simulink model "Control2_exec_time_sampling_time"  (R2023b)
settings: Solver=ode45  StartTime=0.0  StopTime=inf  RelTol=1e-3  EnableMultiTasking=on
libraries: instrumentseriallib x3
settings Model: Creator=fvg  LastModifiedBy=Usuario
settings SolverCC: AlgebraicLoopSolver=TrustRegion
settings DataIOCC: LimitDataPoints=on  SaveFormat=Array  SignalLoggingSaveFormat=ModelDataLogs  SaveTime=off  ReturnWorkspaceOutputs=off
settings OptimizationCC: ExpressionDepthLimit=2147483647  LifeSpan=inf
settings DebuggingCC: UnderspecifiedInitializationDetection=Classic  MergeDetectMultiDrivingBlocksExec=none  SolverPrmCheckMsg=warning  FcnCallInpInsideContextMsg=warning  UnconnectedInputMsg=warning  UnconnectedOutputMsg=warning  UnconnectedLineMsg=warning  StateNameClashWarn=warning  SFUnexpectedBacktrackingDiag=warning  SFNoUnconditionalDefaultTransitionDiag=warning  SFExecutionAtInitializationDiag=none  ArithmeticOperatorsInVariantConditions=warning
settings HardwareCC: ProdBitPerPointer=32  ProdBitPerSizeT=32  ProdBitPerPtrDiffT=32  ProdLargestAtomicFloat=None  ProdIntDivRoundTo=Undefined  ProdEndianess=Unspecified  ProdWordSize=32  ProdHWDeviceType=32-bit Generic
settings ModelReferenceCC: EnableRefExpFcnMdlSchedulingChecks=on  PropagateSignalLabelsOutOfModel=off
settings SFSimCC: SimUseLocalCustomCode=off  CustomCodeUndefinedFunction=UseInterfaceOnly
settings RTWCC: RTWUseLocalCustomCode=off
settings CodeAppCC: StateflowObjectComments=on
settings GRTTargetCC: TargetLangStandard=C89/C90 (ANSI)  CombineOutputUpdateFcns=off  GRTInterface=on
settings ConfigComp: CovMetricSettings=dw  CovSaveCumulativeToWorkspaceVar=on  CovSaveSingleToWorkspaceVar=on  CovExternalEMLEnable=off

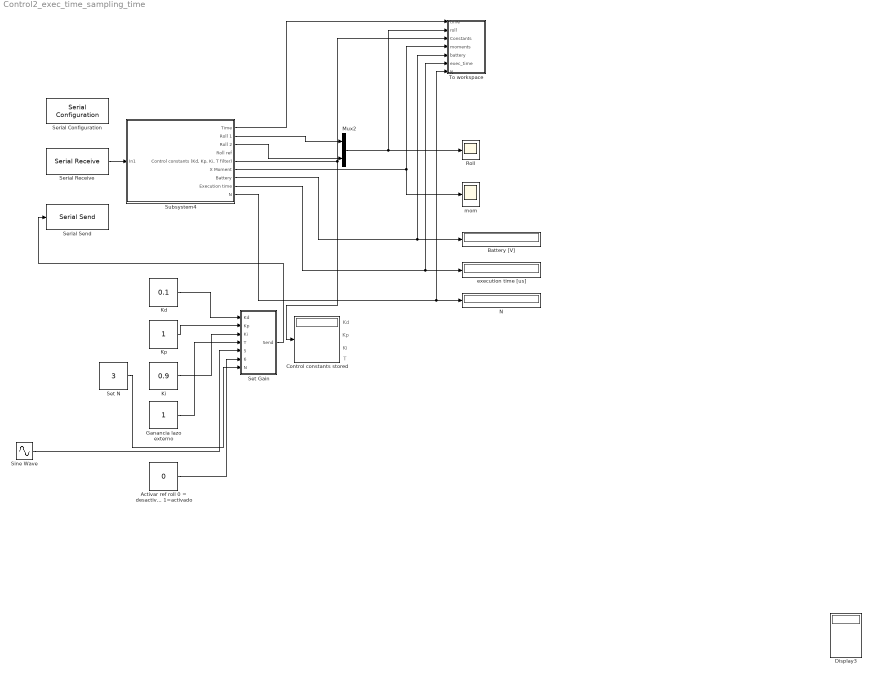
== system Control2_exec_time_sampling_time ==
  note: T
  note: Ki
  note: Kp
  note: Kd
  Activar ref roll 0 = desactivado 1=activado : Constant  Value=0
  Battery [V] : Display
  Control constants stored : Display
  Display3 : Display
  "Ganancia lazo externo " : Constant
  Kd : Constant  Value=0.1
  Ki : Constant  Value=0.9
  Kp : Constant
  Mux2 : Mux  Inputs=2
  N : Display
  Roll : Scope
  Serial Configuration : instrumentseriallib/Serial Configuration  Priority=-200000  PortSel=COM6  Port=COM6  ComPort=COM6  BaudRate=57600  DataBits=8  Parity=none  StopBits=1  ByteOrder=little-endian  FlowControl=none  Timeout=10  SimulateUsing=Interpreted execution  BlockInModel=on  aMode=1
  Serial Receive : instrumentseriallib/Serial Receive  PortSel=COM6  Port=COM6  ComPort=COM6  DataType=uint8  SaveDataType=uint8  ToggleHeader=on  Header="[ 97   98   99  100 ]"  DataSize="[44   1]"  ToggleTerminator=on  Terminator=<none>  CustomTerminator=[]  InputFormat=Column major  ToggleDataSize=on  EnableBlockingMode=on  ActionDataUnavailable=Output last received value  ActionWhenDataUnavailable=Output last received value  CustomValue=0  SampleTime=-1  SimulateUsing=Interpreted execution  BlockInModel=on  aMode=1
  Serial Send : instrumentseriallib/Serial Send  PortSel=COM6  Port=COM6  ComPort=COM6  Header=[]  Terminator=<none>  CustomTerminator=[]  EnableBlockingMode=off  SimulateUsing=Interpreted execution  BlockInModel=on  aMode=1
  Set Gain : Subsystem
  Set N : Constant  Value=3  OutMin=[1]  OutMax=[100]
  Sine Wave : Sin  Amplitude=0.2  Frequency=0.5  SampleTime=0
  Subsystem4 : Subsystem
  "To workspace " : Subsystem
  execution time [us] : Display
  mom : Scope
  wires:
  Kd/1 -> Set Gain/1(Kd)
  Kp/1 -> Set Gain/2(Kp)
  Ki/1 -> Set Gain/3(Ki)
  "Ganancia lazo externo "/1 -> Set Gain/4(T)
  Set Gain/1(Send) -> Serial Send/1
  Mux2/1 -> "To workspace "/2(roll), Roll/1
  Serial Receive/1 -> Subsystem4/1(In1)
  Subsystem4/7(Battery) -> "To workspace "/5(battery), Battery [V]/1
  Subsystem4/2(Roll 1) -> Mux2/1
  Subsystem4/5("Control constants (Kd, Kp, Ki, T filter)") -> Control constants stored/1, "To workspace "/3(Constants)
  Subsystem4/6(X Moment) -> mom/1, "To workspace "/4("moments ")
  Subsystem4/1(Time) -> "To workspace "/1(time)
  Sine Wave/1 -> Set Gain/5(Ref roll)
  Activar ref roll 0 = desactivado 1=activado/1 -> Set Gain/6(Ref roll act)
  Subsystem4/3(Roll 2) -> Mux2/2
  Subsystem4/8(Execution time) -> "To workspace "/6(exec_time), execution time [us]/1
  Subsystem4/9(N) -> "To workspace "/7(N), N/1
  Set N/1 -> Set Gain/7(N)

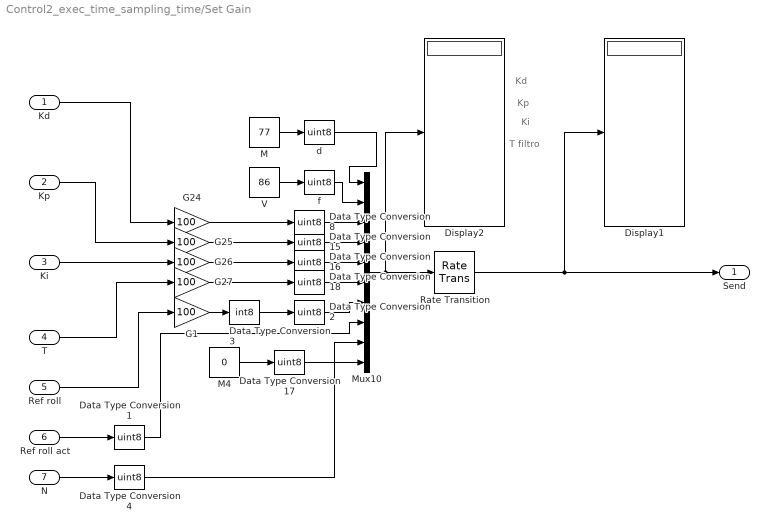
== system Control2_exec_time_sampling_time/Set Gain ==
  note: T filtro
  note: Ki
  note: Kp
  note: Kd
  Kd : Inport
  Kp : Inport  Port=2
  Ki : Inport  Port=3
  T : Inport  Port=4
  Ref roll : Inport  Port=5
  Ref roll act : Inport  Port=6
  N : Inport  Port=7
  Data Type Conversion{1..2,4,8,15..18} (8 alike) : DataTypeConversion  OutDataTypeStr=uint8  SaturateOnIntegerOverflow=off  RndMeth=Floor
  Data Type Conversion3 : DataTypeConversion  OutDataTypeStr=int8  SaturateOnIntegerOverflow=off  RndMeth=Floor
  Display1 : Display
  Display2 : Display
  G{1,24..27} (5 alike) : Gain  Gain=100
  M : Constant  Value=77
  M4 : Constant  Value=0
  Mux10 : Mux  Inputs=10
  Rate Transition : RateTransition  Integrity=off  Deterministic=off  OutPortSampleTime=1
  V : Constant  Value=86
  d : DataTypeConversion  OutDataTypeStr=uint8  SaturateOnIntegerOverflow=off  RndMeth=Floor
  f : DataTypeConversion  OutDataTypeStr=uint8  SaturateOnIntegerOverflow=off  RndMeth=Floor
  Send : Outport  VectorParamsAs1DForOutWhenUnconnected=off
  wires:
  G24/1 -> Data Type Conversion8/1
  Data Type Conversion16/1 -> Mux10/5
  G27/1 -> Data Type Conversion18/1
  G26/1 -> Data Type Conversion16/1
  T/1 -> G27/1
  G25/1 -> Data Type Conversion15/1
  Data Type Conversion8/1 -> Mux10/3
  f/1 -> Mux10/2
  Data Type Conversion18/1 -> Mux10/6
  Data Type Conversion15/1 -> Mux10/4
  Data Type Conversion17/1 -> Mux10/10
  d/1 -> Mux10/1
  Mux10/1 -> Display2/1, Rate Transition/1
  M4/1 -> Data Type Conversion17/1
  Kd/1 -> G24/1
  Kp/1 -> G25/1
  Ki/1 -> G26/1
  V/1 -> f/1
  M/1 -> d/1
  Rate Transition/1 -> Display1/1, Send/1
  Ref roll/1 -> G1/1
  Ref roll act/1 -> Data Type Conversion1/1
  G1/1 -> Data Type Conversion3/1
  Data Type Conversion1/1 -> Mux10/8
  Data Type Conversion2/1 -> Mux10/7
  Data Type Conversion3/1 -> Data Type Conversion2/1
  N/1 -> Data Type Conversion4/1
  Data Type Conversion4/1 -> Mux10/9

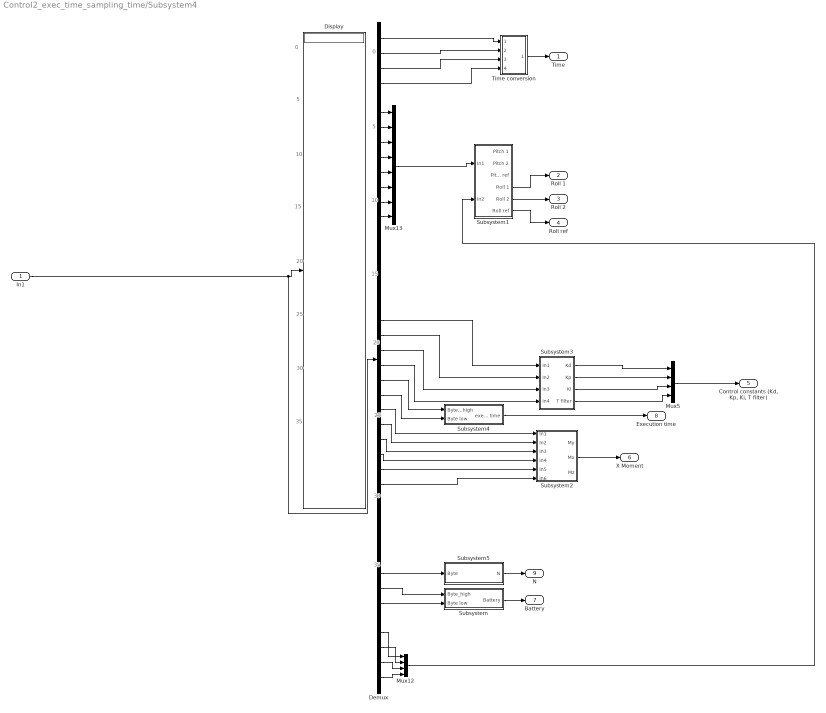
== system Control2_exec_time_sampling_time/Subsystem4 ==
  note: 35
  note: 30
  note: 25
  note: 20
  note: 15
  note: 10
  note: 5
  note: 0
  note: 35
  note: 30
  note: 25
  note: 20
  note: 15
  note: 10
  note: 5
  note: 0
  In1 : Inport
  Demux : Demux  Outputs=44
  Display : Display
  Mux12 : Mux
  Mux13 : Mux  Inputs=8
  Mux5 : Mux
  Subsystem : Subsystem
  Subsystem1 : Subsystem
  Subsystem2 : Subsystem
  Subsystem3 : Subsystem
  Subsystem4 : Subsystem
  Subsystem5 : Subsystem
  Time conversion : Subsystem
  Time : Outport  VectorParamsAs1DForOutWhenUnconnected=off
  Roll 1 : Outport  Port=2  VectorParamsAs1DForOutWhenUnconnected=off
  Roll 2 : Outport  Port=3  VectorParamsAs1DForOutWhenUnconnected=off
  Roll ref : Outport  Port=4  VectorParamsAs1DForOutWhenUnconnected=off
  "Control constants (Kd, Kp, Ki, T filter)" : Outport  Port=5  VectorParamsAs1DForOutWhenUnconnected=off
  X Moment : Outport  Port=6  VectorParamsAs1DForOutWhenUnconnected=off
  Battery : Outport  Port=7  VectorParamsAs1DForOutWhenUnconnected=off
  Execution time : Outport  Port=8  VectorParamsAs1DForOutWhenUnconnected=off
  N : Outport  Port=9  VectorParamsAs1DForOutWhenUnconnected=off
  wires:
  In1/1 -> Display/1, Demux/1
  Subsystem1/4(Roll 1) -> Roll 1/1
  Mux13/1 -> Subsystem1/1(In1)
  Subsystem1/5(Roll 2) -> Roll 2/1
  Subsystem1/6(Roll ref) -> Roll ref/1
  Mux12/1 -> Subsystem1/2(In2)
  Demux/39 -> Subsystem/2(Byte low)
  Time conversion/1(Time) -> Time/1
  Demux/4 -> Time conversion/4(In4)
  Demux/3 -> Time conversion/3(In3)
  Demux/2 -> Time conversion/2(In2)
  Demux/1 -> Time conversion/1(In1)
  Demux/30 -> Subsystem2/5(In5)
  Demux/29 -> Subsystem2/4(In4)
  Demux/26 -> Subsystem2/1(In1)
  Demux/31 -> Subsystem2/6(In6)
  Demux/28 -> Subsystem2/3(In3)
  Demux/27 -> Subsystem2/2(In2)
  Demux/9 -> Mux13/4
  Demux/10 -> Mux13/5
  Demux/8 -> Mux13/3
  Mux5/1 -> "Control constants (Kd, Kp, Ki, T filter)"/1
  Demux/6 -> Mux13/1
  Demux/12 -> Mux13/7
  Demux/13 -> Mux13/8
  Demux/42 -> Mux12/2
  Demux/41 -> Mux12/1
  Demux/11 -> Mux13/6
  Demux/7 -> Mux13/2
  Demux/44 -> Mux12/4
  Demux/43 -> Mux12/3
  Subsystem3/4(T filter) -> Mux5/4
  Demux/23 -> Subsystem3/4(In4)
  Subsystem3/1(Kd) -> Mux5/1
  Demux/22 -> Subsystem3/3(In3)
  Subsystem2/2(Mx) -> X Moment/1
  Subsystem3/3(Ki) -> Mux5/3
  Subsystem3/2(Kp) -> Mux5/2
  Demux/20 -> Subsystem3/1(In1)
  Demux/21 -> Subsystem3/2(In2)
  Subsystem/1(Battery) -> Battery/1
  Demux/38 -> Subsystem/1(Byte_high)
  Demux/24 -> Subsystem4/1(Byte_high)
  Demux/25 -> Subsystem4/2(Byte low)
  Subsystem4/1(exec time) -> Execution time/1
  Subsystem5/1(N) -> N/1
  Demux/37 -> Subsystem5/1(Byte)

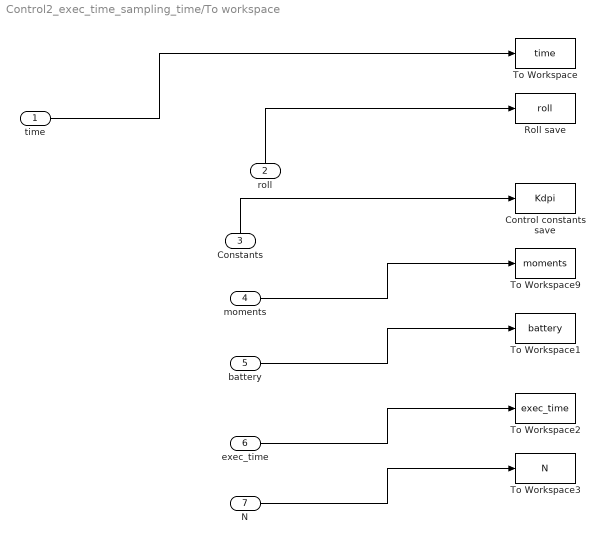
== system Control2_exec_time_sampling_time/To workspace  ==
  time : Inport
  roll : Inport  Port=2
  Constants : Inport  Port=3
  "moments " : Inport  Port=4
  battery : Inport  Port=5
  exec_time : Inport  Port=6
  N : Inport  Port=7
  Control constants save : ToWorkspace  VariableName=Kdpi  SampleTime=-1
  Roll save : ToWorkspace  VariableName=roll  SampleTime=-1
  To Workspace : ToWorkspace  VariableName=time  SampleTime=-1
  To Workspace1 : ToWorkspace  VariableName=battery  SampleTime=-1
  To Workspace2 : ToWorkspace  VariableName=exec_time  SampleTime=-1
  To Workspace3 : ToWorkspace  VariableName=N  SampleTime=-1
  To Workspace9 : ToWorkspace  VariableName=moments  SampleTime=-1
  wires:
  time/1 -> To Workspace/1
  roll/1 -> Roll save/1
  Constants/1 -> Control constants save/1
  "moments "/1 -> To Workspace9/1
  battery/1 -> To Workspace1/1
  exec_time/1 -> To Workspace2/1
  N/1 -> To Workspace3/1

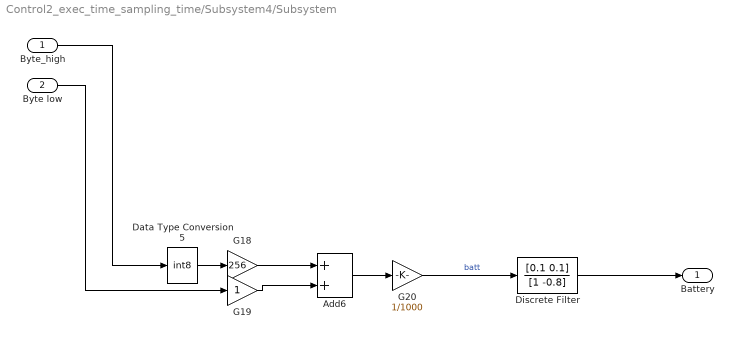
== system Control2_exec_time_sampling_time/Subsystem4/Subsystem ==
  Byte_high : Inport
  Byte low : Inport  Port=2
  Add6 : Sum
  Data Type Conversion5 : DataTypeConversion  OutDataTypeStr=int8  SaturateOnIntegerOverflow=off  RndMeth=Floor
  Discrete Filter : DiscreteFilter  Numerator=[0.1 0.1]  Denominator=[1 -0.8]  InitialStates=60  SampleTime=0.05
  G18 : Gain  Gain=256
  G19 : Gain
  G20 : Gain  Gain=1/1000
  Battery : Outport  VectorParamsAs1DForOutWhenUnconnected=off
  wires:
  Byte low/1 -> G19/1
  Discrete Filter/1 -> Battery/1
  Byte_high/1 -> Data Type Conversion5/1
  G18/1 -> Add6/1
  G20/1 -> Discrete Filter/1  "batt"
  Data Type Conversion5/1 -> G18/1
  G19/1 -> Add6/2
  Add6/1 -> G20/1

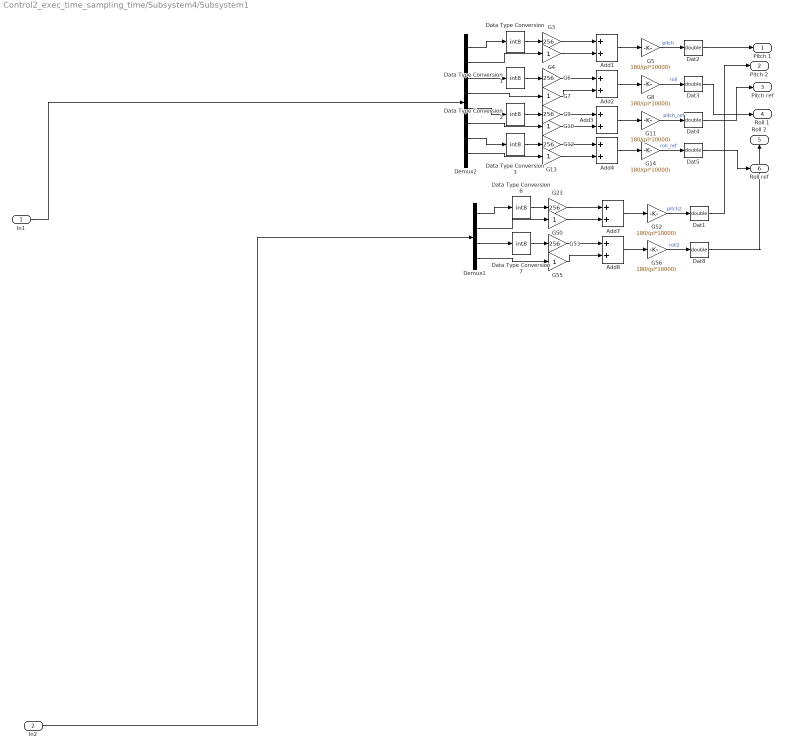
== system Control2_exec_time_sampling_time/Subsystem4/Subsystem1 ==
  In1 : Inport
  In2 : Inport  Port=2
  Add{1..4,7..8} (6 alike) : Sum
  Dat{1..5,8} (6 alike) : DataTypeConversion  OutDataTypeStr=double  RndMeth=Simplest  SaturateOnIntegerOverflow=off
  Data Type Conversion{,1..3,6..7} (6 alike) : DataTypeConversion  OutDataTypeStr=int8  SaturateOnIntegerOverflow=off  RndMeth=Floor
  Demux1 : Demux
  Demux2 : Demux  Outputs=8
  G{4,7,10,13,50,55} (6 alike) : Gain
  G{5,8,11,14,52,56} (6 alike) : Gain  Gain=180/(pi*10000)
  G{3,6,9,12,23,53} (6 alike) : Gain  Gain=256
  Pitch 1 : Outport  VectorParamsAs1DForOutWhenUnconnected=off
  Pitch 2 : Outport  Port=2  VectorParamsAs1DForOutWhenUnconnected=off
  Pitch ref : Outport  Port=3  VectorParamsAs1DForOutWhenUnconnected=off
  Roll 1 : Outport  Port=4  VectorParamsAs1DForOutWhenUnconnected=off
  Roll 2 : Outport  Port=5  VectorParamsAs1DForOutWhenUnconnected=off
  Roll ref : Outport  Port=6  VectorParamsAs1DForOutWhenUnconnected=off
  wires:
  Dat4/1 -> Pitch ref/1
  Dat3/1 -> Roll 1/1
  Dat2/1 -> Pitch 1/1
  Dat5/1 -> Roll ref/1
  Add2/1 -> G8/1
  Add4/1 -> G14/1
  G7/1 -> Add2/2
  G12/1 -> Add4/1
  Data Type Conversion2/1 -> G9/1
  Add3/1 -> G11/1
  G10/1 -> Add3/2
  G9/1 -> Add3/1
  Data Type Conversion1/1 -> G6/1
  G13/1 -> Add4/2
  G11/1 -> Dat4/1  "pitch_ref"
  G14/1 -> Dat5/1  "roll_ref"
  G5/1 -> Dat2/1  "pitch"
  G3/1 -> Add1/1
  G4/1 -> Add1/2
  Add1/1 -> G5/1
  Data Type Conversion/1 -> G3/1
  G6/1 -> Add2/1
  Data Type Conversion3/1 -> G12/1
  G8/1 -> Dat3/1  "roll"
  In2/1 -> Demux1/1
  Demux1/3 -> Data Type Conversion7/1
  Demux2/8 -> G13/1
  G56/1 -> Dat8/1  "roll2"
  Demux1/1 -> Data Type Conversion6/1
  Demux1/2 -> G50/1
  In1/1 -> Demux2/1
  Demux2/1 -> Data Type Conversion/1
  Dat8/1 -> Roll 2/1
  Demux1/4 -> G55/1
  Add8/1 -> G56/1
  Data Type Conversion7/1 -> G53/1
  Demux2/6 -> G10/1
  G52/1 -> Dat1/1  "pitch2"
  G55/1 -> Add8/2
  Demux2/7 -> Data Type Conversion3/1
  G23/1 -> Add7/1
  Add7/1 -> G52/1
  Data Type Conversion6/1 -> G23/1
  G50/1 -> Add7/2
  G53/1 -> Add8/1
  Dat1/1 -> Pitch 2/1
  Demux2/5 -> Data Type Conversion2/1
  Demux2/2 -> G4/1
  Demux2/3 -> Data Type Conversion1/1
  Demux2/4 -> G7/1

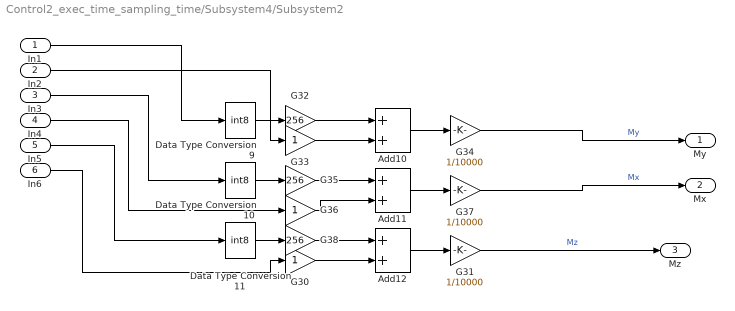
== system Control2_exec_time_sampling_time/Subsystem4/Subsystem2 ==
  In1 : Inport
  In2 : Inport  Port=2
  In3 : Inport  Port=3
  In4 : Inport  Port=4
  In5 : Inport  Port=5
  In6 : Inport  Port=6
  Add10 : Sum
  Add11 : Sum
  Add12 : Sum
  Data Type Conversion10 : DataTypeConversion  OutDataTypeStr=int8  SaturateOnIntegerOverflow=off  RndMeth=Floor
  Data Type Conversion11 : DataTypeConversion  OutDataTypeStr=int8  SaturateOnIntegerOverflow=off  RndMeth=Floor
  Data Type Conversion9 : DataTypeConversion  OutDataTypeStr=int8  SaturateOnIntegerOverflow=off  RndMeth=Floor
  G30 : Gain
  G31 : Gain  Gain=1/10000
  G32 : Gain  Gain=256
  G33 : Gain
  G34 : Gain  Gain=1/10000
  G35 : Gain  Gain=256
  G36 : Gain
  G37 : Gain  Gain=1/10000
  G38 : Gain  Gain=256
  My : Outport  VectorParamsAs1DForOutWhenUnconnected=off
  Mx : Outport  Port=2  VectorParamsAs1DForOutWhenUnconnected=off
  Mz : Outport  Port=3  VectorParamsAs1DForOutWhenUnconnected=off
  wires:
  G33/1 -> Add10/2
  Data Type Conversion10/1 -> G35/1
  G38/1 -> Add12/1
  G32/1 -> Add10/1
  Add11/1 -> G37/1
  Data Type Conversion9/1 -> G32/1
  G35/1 -> Add11/1
  G36/1 -> Add11/2
  Add10/1 -> G34/1
  G31/1 -> Mz/1  "Mz"
  G37/1 -> Mx/1  "Mx"
  In2/1 -> G33/1
  In3/1 -> Data Type Conversion10/1
  In5/1 -> Data Type Conversion11/1
  In1/1 -> Data Type Conversion9/1
  In6/1 -> G30/1
  In4/1 -> G36/1
  Data Type Conversion11/1 -> G38/1
  G30/1 -> Add12/2
  Add12/1 -> G31/1
  G34/1 -> My/1  "My"

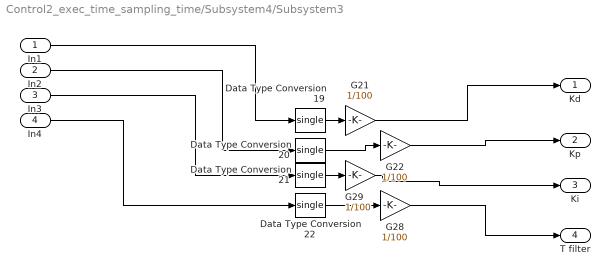
== system Control2_exec_time_sampling_time/Subsystem4/Subsystem3 ==
  In1 : Inport
  In2 : Inport  Port=2
  In3 : Inport  Port=3
  In4 : Inport  Port=4
  Data Type Conversion{19..22} (4 alike) : DataTypeConversion  OutDataTypeStr=single  SaturateOnIntegerOverflow=off  RndMeth=Floor
  G{21..22,28..29} (4 alike) : Gain  Gain=1/100
  Kd : Outport  VectorParamsAs1DForOutWhenUnconnected=off
  Kp : Outport  Port=2  VectorParamsAs1DForOutWhenUnconnected=off
  Ki : Outport  Port=3  VectorParamsAs1DForOutWhenUnconnected=off
  T filter : Outport  Port=4  VectorParamsAs1DForOutWhenUnconnected=off
  wires:
  In1/1 -> Data Type Conversion19/1
  In3/1 -> Data Type Conversion21/1
  Data Type Conversion20/1 -> G22/1
  Data Type Conversion19/1 -> G21/1
  G29/1 -> Ki/1
  G28/1 -> T filter/1
  In4/1 -> Data Type Conversion22/1
  Data Type Conversion22/1 -> G28/1
  Data Type Conversion21/1 -> G29/1
  In2/1 -> Data Type Conversion20/1
  G21/1 -> Kd/1
  G22/1 -> Kp/1

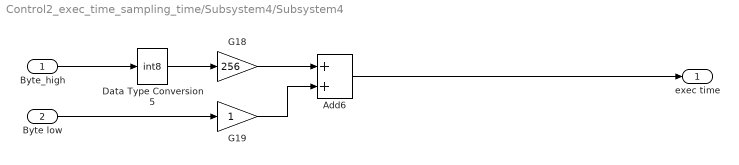
== system Control2_exec_time_sampling_time/Subsystem4/Subsystem4 ==
  Byte_high : Inport
  Byte low : Inport  Port=2
  Add6 : Sum
  Data Type Conversion5 : DataTypeConversion  OutDataTypeStr=int8  SaturateOnIntegerOverflow=off  RndMeth=Floor
  G18 : Gain  Gain=256
  G19 : Gain
  exec time : Outport  VectorParamsAs1DForOutWhenUnconnected=off
  wires:
  Byte low/1 -> G19/1
  Add6/1 -> exec time/1
  Byte_high/1 -> Data Type Conversion5/1
  G18/1 -> Add6/1
  Data Type Conversion5/1 -> G18/1
  G19/1 -> Add6/2

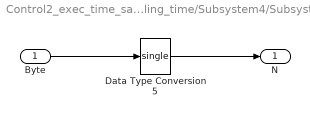
== system Control2_exec_time_sampling_time/Subsystem4/Subsystem5 ==
  Byte : Inport
  Data Type Conversion5 : DataTypeConversion  OutDataTypeStr=single  SaturateOnIntegerOverflow=off  RndMeth=Floor
  N : Outport  VectorParamsAs1DForOutWhenUnconnected=off
  wires:
  Byte/1 -> Data Type Conversion5/1
  Data Type Conversion5/1 -> N/1

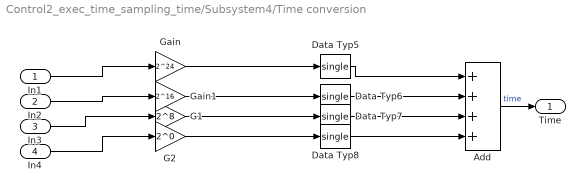
== system Control2_exec_time_sampling_time/Subsystem4/Time conversion ==
  In1 : Inport
  In2 : Inport  Port=2
  In3 : Inport  Port=3
  In4 : Inport  Port=4
  Add : Sum  Inputs=++++
  Data Typ{5..8} (4 alike) : DataTypeConversion  OutDataTypeStr=single  SaturateOnIntegerOverflow=off  RndMeth=Floor
  G1 : Gain  Gain=2^8
  G2 : Gain  Gain=2^0
  Gain : Gain  Gain=2^24
  Gain1 : Gain  Gain=2^16
  Time : Outport  VectorParamsAs1DForOutWhenUnconnected=off
  wires:
  Data Typ5/1 -> Add/1
  In3/1 -> G1/1
  Data Typ7/1 -> Add/3
  Data Typ8/1 -> Add/4
  Data Typ6/1 -> Add/2
  In2/1 -> Gain1/1
  G2/1 -> Data Typ8/1
  Add/1 -> Time/1  "time"
  In1/1 -> Gain/1
  In4/1 -> G2/1
  Gain/1 -> Data Typ5/1
  G1/1 -> Data Typ7/1
  Gain1/1 -> Data Typ6/1
